simulink model "simulink_prob"  (R2024a)
settings: Solver=VariableStepAuto  StartTime=0.0  StopTime=1  RelTol=1e-3
values from neighbouring files (symbols this model uses):
  c = 340    [APP4.m]    (also in APP4_automated.m; APP4_automated2.m)
  d = 1    [APP4.m]    (also in APP4_automated.m; APP4_automated2.m)
undefined symbols (not defined in the file or in its folder): elec_den_coefs_Fostex, elec_den_coefs_SEAS, elec_num_coefs_Fostex, elec_num_coefs_SEAS, global_den_coefs_Fostex, global_den_coefs_SEAS, global_num_coefs_Fostex, global_num_coefs_SEAS
settings Model: Creator=boum0704  LastModifiedBy=boum0704

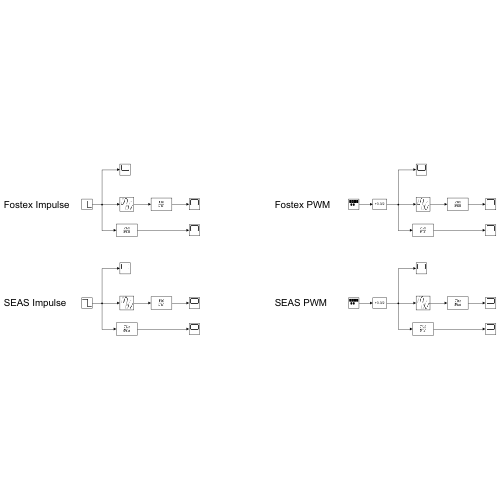
[thumbnail: Simulink's stored preview of the top-level diagram]
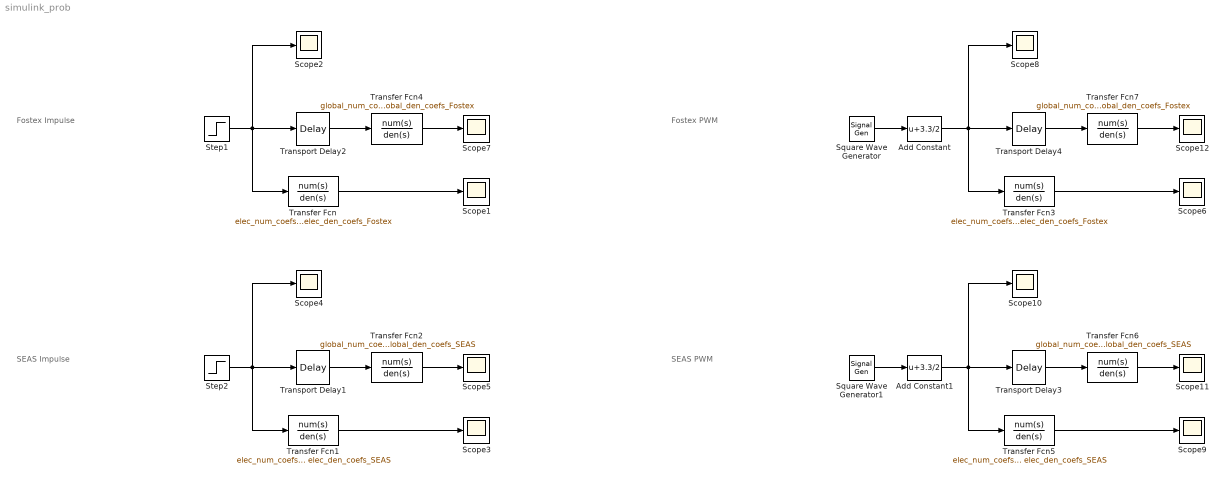
== system simulink_prob ==
  note: Fostex Impulse
  note: SEAS Impulse
  note: Fostex PWM
  note: SEAS PWM
  Add Constant : Bias  Bias=3.3/2  SaturateOnIntegerOverflow=off
  Add Constant1 : Bias  Bias=3.3/2  SaturateOnIntegerOverflow=off
  Scope{1..12} (12 alike) : Scope
  Square Wave Generator : SignalGenerator  WaveForm=square  Amplitude=3.3/2  Frequency=100
  Square Wave Generator1 : SignalGenerator  WaveForm=square  Amplitude=3.3/2  Frequency=100
  Step1 : Step  Time=0.01  Before=3.3  After=0  SampleTime=0  VectorParams1D=off  ZeroCross=off
  Step2 : Step  Time=0.01  Before=3.3  After=0  SampleTime=0  VectorParams1D=off  ZeroCross=off
  Transfer Fcn : TransferFcn  Numerator=elec_num_coefs_Fostex  Denominator=elec_den_coefs_Fostex  ContinuousStateAttributes='He'
  Transfer Fcn1 : TransferFcn  Numerator=elec_num_coefs_SEAS  Denominator=elec_den_coefs_SEAS  ContinuousStateAttributes='He'
  Transfer Fcn2 : TransferFcn  Numerator=global_num_coefs_SEAS  Denominator=global_den_coefs_SEAS  ContinuousStateAttributes='He'
  Transfer Fcn3 : TransferFcn  Numerator=elec_num_coefs_Fostex  Denominator=elec_den_coefs_Fostex  ContinuousStateAttributes='He'
  Transfer Fcn4 : TransferFcn  Numerator=global_num_coefs_Fostex  Denominator=global_den_coefs_Fostex  ContinuousStateAttributes='He'
  Transfer Fcn5 : TransferFcn  Numerator=elec_num_coefs_SEAS  Denominator=elec_den_coefs_SEAS  ContinuousStateAttributes='He'
  Transfer Fcn6 : TransferFcn  Numerator=global_num_coefs_SEAS  Denominator=global_den_coefs_SEAS  ContinuousStateAttributes='He'
  Transfer Fcn7 : TransferFcn  Numerator=global_num_coefs_Fostex  Denominator=global_den_coefs_Fostex  ContinuousStateAttributes='He'
  Transport Delay{1..4} (4 alike) : TransportDelay  DelayTime=d/c  BufferSize=2048  TransDelayFeedthrough=on
  wires:
  Step1/1 -> Scope2/1, Transfer Fcn/1, Transport Delay2/1
  Transfer Fcn/1 -> Scope1/1
  Transfer Fcn4/1 -> Scope7/1
  Transport Delay2/1 -> Transfer Fcn4/1
  Transport Delay1/1 -> Transfer Fcn2/1
  Transfer Fcn2/1 -> Scope5/1
  Transfer Fcn1/1 -> Scope3/1
  Step2/1 -> Transport Delay1/1, Transfer Fcn1/1, Scope4/1
  Add Constant1/1 -> Scope10/1, Transfer Fcn5/1, Transport Delay3/1
  Transfer Fcn5/1 -> Scope9/1
  Transfer Fcn6/1 -> Scope11/1
  Transport Delay3/1 -> Transfer Fcn6/1
  Transport Delay4/1 -> Transfer Fcn7/1
  Transfer Fcn7/1 -> Scope12/1
  Transfer Fcn3/1 -> Scope6/1
  Add Constant/1 -> Transport Delay4/1, Transfer Fcn3/1, Scope8/1
  Square Wave Generator/1 -> Add Constant/1
  Square Wave Generator1/1 -> Add Constant1/1
